simulink model "Test_Plain_SPI_Transfer"  (R2018a)
settings: Solver=FixedStepAuto  StartTime=0.0  StopTime=inf  FixedStep=.015  RelTol=1e-3  EnableMultiTasking=on
libraries: raspberrypilib x2, simulink x1
settings Model: SimulationMode=external  Creator=domin  LastModifiedBy=domin
settings SolverCC: PositivePriorityOrder=on  AutoInsertRateTranBlk=on
settings OptimizationCC: EnhancedBackFolding=on  PassReuseOutputArgsThreshold=0  MaxStackSize=64  OptimizeBlockOrder=speed  DifferentSizesBufferReuse=on  OptimizationCustomize=off
settings DebuggingCC: ParameterTunabilityLossMsg=error
settings HardwareCC: ProdBitPerPointer=32  ProdBitPerSizeT=32  ProdBitPerPtrDiffT=32  ProdLargestAtomicInteger=Long  ProdLargestAtomicFloat=Double  ProdWordSize=32  ProdHWDeviceType=ARM Compatible->ARM Cortex  UseEmbeddedCoderFeatures=off
settings SFSimCC: MATLABDynamicMemAlloc=off
settings RTWCC: SystemTargetFile=ert.tlc  HardwareBoard=Raspberry Pi  TLCOptions="-aInlineSetEventsForThisBaseRateFcn=TLC_FALSE -aSuppressMultiTaskScheduler=TLC_FALSE  -aRateBasedStepFcn=0"  TemplateMakefile=ert_default_tmf  GenerateReport=on  Toolchain=GNU GCC Raspberry Pi  BuildConfiguration=Faster Runs  LaunchReport=on
settings CodeAppCC: ForceParamTrailComments=on  OperatorAnnotations=on
settings ERTTargetCC: ERTCustomFileBanners=off  SupportContinuousTime=on  SupportNonInlinedSFcns=on  RemoveResetFunc=off  SupportVariableSizeSignals=on  ModelStepFunctionPrototypeControlCompliant=off

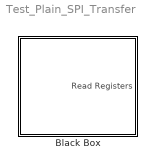
== system Test_Plain_SPI_Transfer ==
  Black Box : Subsystem

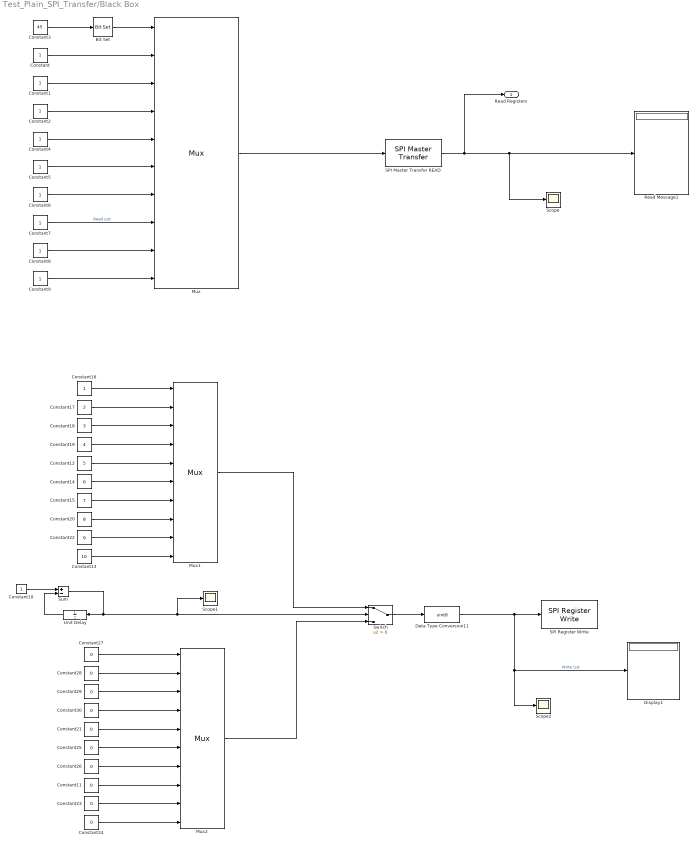
== system Test_Plain_SPI_Transfer/Black Box ==
  Bit Set : simulink/Logic and Bit Operations/Bit Set  iBit=7
      settings: SourceProductName=Simulink  SourceProductBaseCode=SL
  Constant{,1..2,4..9} (9 alike) : Constant  OutDataTypeStr=uint8
  Constant10 : Constant
  Constant{11,21,23..30} (10 alike) : Constant  Value=0
  Constant12 : Constant  Value=5
  Constant13 : Constant  Value=10
  Constant14 : Constant  Value=6
  Constant15 : Constant  Value=7
  Constant16 : Constant
  Constant17 : Constant  Value=2
  Constant18 : Constant  Value=3
  Constant19 : Constant  Value=4
  Constant20 : Constant  Value=8
  Constant22 : Constant  Value=9
  Constant3 : Constant  Value=45  OutDataTypeStr=uint8
  Data Type Conversion11 : DataTypeConversion  OutDataTypeStr=uint8  SaturateOnIntegerOverflow=on
  Display1 : Display
      settings: Format=binary (Stored Integer)
  Mux : Mux  Inputs=10
      settings: DisplayOption=signals
  Mux1 : Mux  Inputs=10
      settings: DisplayOption=signals
  Mux2 : Mux  Inputs=10
      settings: DisplayOption=signals
  Read Message1 : Display
      settings: Format=decimal (Stored Integer)
  SPI Master Transfer READ : raspberrypilib/SPI Master Transfer  BoardProperty=Pi 3 Model B  SPIModule=uint32(0)  Mode=Master  BusSpeed=1000000  Pin=SPI0_CE1  FirstBitToTransfer=Most significant bit (MSB)  ClockMode=0  BlockFunction=Transfer  RegisterAddress=0  OutputDataType=int8  OutputDataLength=1
      settings: SourceProductName=Simulink Support Package for Raspberry Pi Hardware  SourceProductBaseCode=RASPPI
  SPI Register Write : raspberrypilib/SPI Register Write  BoardProperty=Pi 3 Model B  SPIModule=uint32(0)  Mode=Master  BusSpeed=1000000  Pin=SPI0_CE1  FirstBitToTransfer=Most significant bit (MSB)  ClockMode=0  BlockFunction=Write  RegisterAddress=45  OutputDataType=int8  OutputDataLength=1
      settings: SourceProductName=Simulink Support Package for Raspberry Pi Hardware  SourceProductBaseCode=RASPPI
  Scope : Scope
  Scope1 : Scope
  Scope2 : Scope
  Sum : Sum  Inputs=+-  SaturateOnIntegerOverflow=on  InputSameDT=on  OutDataTypeStr=Inherit: Same as first input
  Switch : Switch  Criteria=u2 > Threshold
  Unit Delay : UnitDelay  SampleTime=-1
  Read Registers : Outport
  wires:
  Constant/1 -> Mux/2
  Bit Set/1 -> Mux/1
  Constant4/1 -> Mux/5
  Data Type Conversion11/1 -> Scope2/1, Display1/1, SPI Register Write/1  "Write List"
  Constant7/1 -> Mux/8  "Read List"
  Constant9/1 -> Mux/10
  Constant3/1 -> Bit Set/1
  Constant1/1 -> Mux/3
  Constant5/1 -> Mux/6
  Constant2/1 -> Mux/4
  Constant8/1 -> Mux/9
  Constant6/1 -> Mux/7
  Mux/1 -> SPI Master Transfer READ/1
  SPI Master Transfer READ/1 -> Read Registers/1, Scope/1, Read Message1/1
  Switch/1 -> Data Type Conversion11/1
  Mux2/1 -> Switch/3
  Constant29/1 -> Mux2/3
  Constant19/1 -> Mux1/4
  Sum/1 -> Unit Delay/1, Scope1/1, Switch/2
  Constant25/1 -> Mux2/6
  Constant27/1 -> Mux2/1
  Constant14/1 -> Mux1/6
  Constant11/1 -> Mux2/8
  Constant21/1 -> Mux2/5
  Mux1/1 -> Switch/1
  Constant22/1 -> Mux1/9
  Constant24/1 -> Mux2/10
  Constant26/1 -> Mux2/7
  Constant10/1 -> Sum/1
  Constant30/1 -> Mux2/4
  Unit Delay/1 -> Sum/2
  Constant28/1 -> Mux2/2
  Constant17/1 -> Mux1/2
  Constant15/1 -> Mux1/7
  Constant12/1 -> Mux1/5
  Constant16/1 -> Mux1/1
  Constant18/1 -> Mux1/3
  Constant13/1 -> Mux1/10
  Constant20/1 -> Mux1/8
  Constant23/1 -> Mux2/9
